simulink model "LaneMaintainSystem_Kavya"  (R2022b)
settings: Solver=VariableStepAuto  StartTime=0.0  StopTime=5  FixedStep=0.01  RelTol=1e-3
values from neighbouring files (symbols this model uses):
  A = [-0.5  -0.3  -0.01; 1  0  0; 0  1  0]    [kavya.mat]
  B = [1 0 0]    [kavya.mat]
  C = [0 0 1]    [kavya.mat]
  Ke = [2.00093781518 12.4255969567 11.1736830953]    [kavya.mat]
  Kr = [14.0661259067 105.961011965 9.990005]    [kavya.mat]
  uD = -0.1    [kavya.mat]
settings Model: Creator=abane  LastModifiedBy=chand

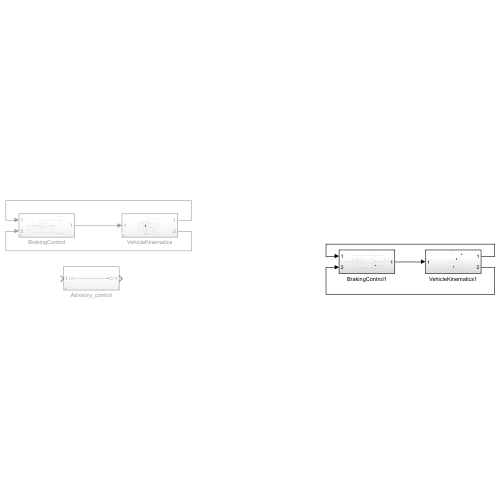
[thumbnail: Simulink's stored preview of the top-level diagram]
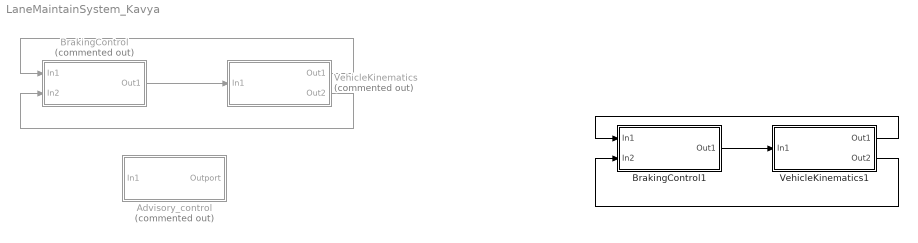
== system LaneMaintainSystem_Kavya ==
  Advisory_control : Subsystem  Commented=on
  BrakingControl : Subsystem  Commented=on
  BrakingControl1 : Subsystem
  VehicleKinematics : Subsystem  Commented=on
  VehicleKinematics1 : Subsystem
  wires:
  BrakingControl/1(Out1) -> VehicleKinematics/1(In1)
  VehicleKinematics/2(Out2) -> BrakingControl/2(In2)
  VehicleKinematics/1(Out1) -> BrakingControl/1(In1)
  BrakingControl1/1(Out1) -> VehicleKinematics1/1(In1)
  VehicleKinematics1/1(Out1) -> BrakingControl1/1(In1)
  VehicleKinematics1/2(Out2) -> BrakingControl1/2(In2)

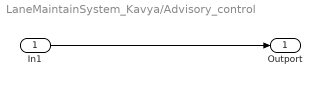
== system LaneMaintainSystem_Kavya/Advisory_control ==
  In1 : Inport
  Outport : Outport
  wires:
  In1/1 -> Outport/1

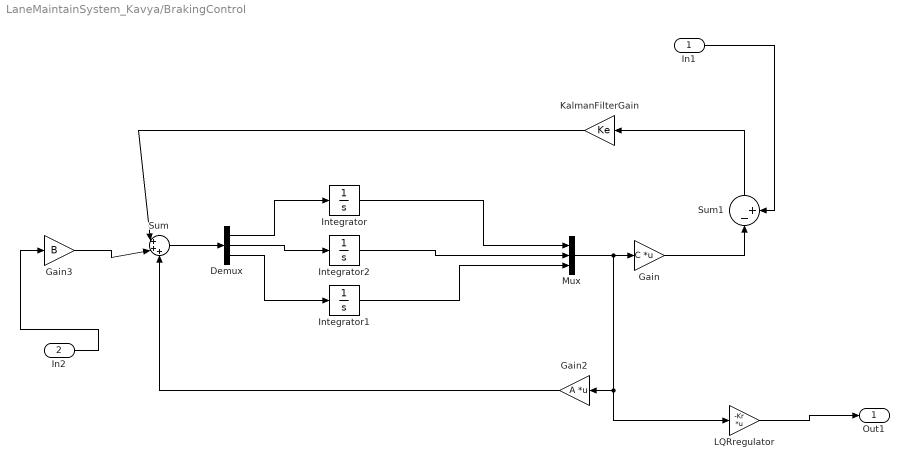
== system LaneMaintainSystem_Kavya/BrakingControl ==
  In1 : Inport
  In2 : Inport  Port=2
  Demux : Demux  Outputs=3
  Gain : Gain  Gain=C  Multiplication=Matrix(K*u)
  Gain2 : Gain  Gain=A  Multiplication=Matrix(K*u)
  Gain3 : Gain  Gain=B
  Integrator : Integrator
  Integrator1 : Integrator
  Integrator2 : Integrator
  KalmanFilterGain : Gain  Gain=Ke
  LQRregulator : Gain  Gain=-Kr  Multiplication=Matrix(K*u)
  Mux : Mux  Inputs=3
  Sum : Sum  Inputs=|+++
  Sum1 : Sum  Inputs=|-+
  Out1 : Outport
  wires:
  Sum/1 -> Demux/1
  Demux/1 -> Integrator/1
  Demux/3 -> Integrator1/1
  Integrator/1 -> Mux/1
  Integrator1/1 -> Mux/3
  Mux/1 -> LQRregulator/1, Gain2/1, Gain/1
  Gain/1 -> Sum1/1
  Sum1/1 -> KalmanFilterGain/1
  KalmanFilterGain/1 -> Sum/1
  Gain2/1 -> Sum/3
  Gain3/1 -> Sum/2
  LQRregulator/1 -> Out1/1
  In2/1 -> Gain3/1
  Demux/2 -> Integrator2/1
  Integrator2/1 -> Mux/2
  In1/1 -> Sum1/2

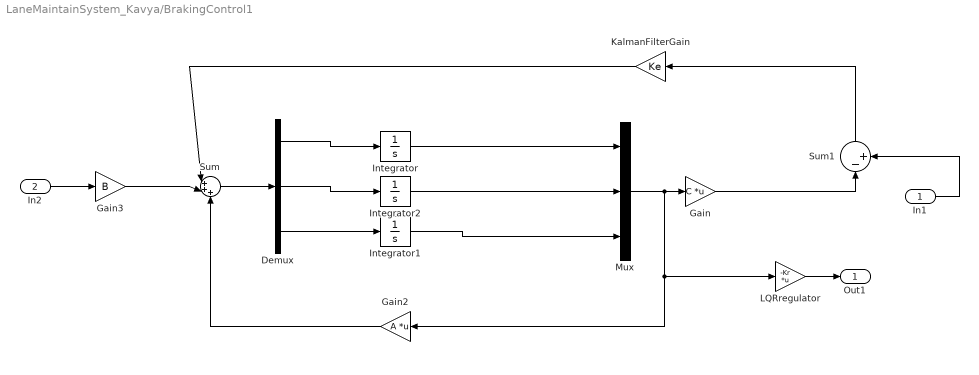
== system LaneMaintainSystem_Kavya/BrakingControl1 ==
  In1 : Inport
  In2 : Inport  Port=2
  Demux : Demux  Outputs=3
  Gain : Gain  Gain=C  Multiplication=Matrix(K*u)
  Gain2 : Gain  Gain=A  Multiplication=Matrix(K*u)
  Gain3 : Gain  Gain=B
  Integrator : Integrator
  Integrator1 : Integrator
  Integrator2 : Integrator
  KalmanFilterGain : Gain  Gain=Ke
  LQRregulator : Gain  Gain=-Kr  Multiplication=Matrix(K*u)
  Mux : Mux  Inputs=3
  Sum : Sum  Inputs=|+++
  Sum1 : Sum  Inputs=|-+
  Out1 : Outport
  wires:
  In1/1 -> Sum1/2
  Integrator2/1 -> Mux/2
  Demux/2 -> Integrator2/1
  In2/1 -> Gain3/1
  LQRregulator/1 -> Out1/1
  Gain3/1 -> Sum/2
  Gain2/1 -> Sum/3
  KalmanFilterGain/1 -> Sum/1
  Sum1/1 -> KalmanFilterGain/1
  Gain/1 -> Sum1/1
  Mux/1 -> Gain2/1, LQRregulator/1, Gain/1
  Integrator1/1 -> Mux/3
  Integrator/1 -> Mux/1
  Demux/3 -> Integrator1/1
  Demux/1 -> Integrator/1
  Sum/1 -> Demux/1

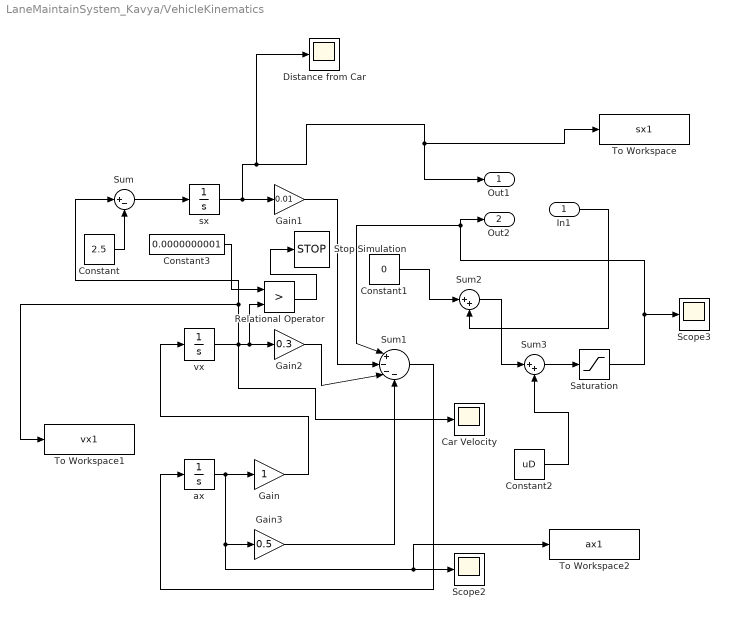
== system LaneMaintainSystem_Kavya/VehicleKinematics ==
  In1 : Inport
  Car Velocity : Scope
  Constant : Constant  Value=2.5
  Constant1 : Constant  Value=0
  Constant2 : Constant  Value=uD
  Constant3 : Constant  Value=0.0000000001
  Distance from Car : Scope
  Gain : Gain
  Gain1 : Gain  Gain=0.01
  Gain2 : Gain  Gain=0.3
  Gain3 : Gain  Gain=0.5
  Relational Operator : RelationalOperator  Operator=>  OutDataTypeStr=boolean  RndMeth=Simplest  InputSameDT=off
  Saturation : Saturate  UpperLimit=0  LowerLimit=-200
  Scope2 : Scope
  Scope3 : Scope
  Stop Simulation : Stop
  Sum : Sum  Inputs=|+-
  Sum1 : Sum  Inputs=|+---
  Sum2 : Sum  Inputs=|++
  Sum3 : Sum  Inputs=|++
  To Workspace : ToWorkspace  VariableName=sx1  SaveFormat=Timeseries  SampleTime=-1
  To Workspace1 : ToWorkspace  VariableName=vx1  SaveFormat=Timeseries  SampleTime=-1
  To Workspace2 : ToWorkspace  VariableName=ax1  SaveFormat=Timeseries  SampleTime=-1
  ax : Integrator
  sx : Integrator  InitialCondition=-43.8
  vx : Integrator  InitialCondition=41.2
  Out1 : Outport
  Out2 : Outport  Port=2
  wires:
  Constant/1 -> Sum/2
  Sum3/1 -> Saturation/1
  Constant2/1 -> Sum3/2
  Gain1/1 -> Sum1/2
  vx/1 -> Car Velocity/1, To Workspace1/1, Sum/1, Relational Operator/2, Gain2/1
  Saturation/1 -> Out2/1, Sum1/1, Scope3/1
  Gain3/1 -> Sum1/4
  Sum1/1 -> ax/1
  sx/1 -> Distance from Car/1, Out1/1, To Workspace/1, Gain1/1
  Sum2/1 -> Sum3/1
  ax/1 -> To Workspace2/1, Scope2/1, Gain3/1, Gain/1
  In1/1 -> Sum2/2
  Gain2/1 -> Sum1/3
  Constant1/1 -> Sum2/1
  Gain/1 -> vx/1
  Sum/1 -> sx/1
  Relational Operator/1 -> Stop Simulation/1
  Constant3/1 -> Relational Operator/1

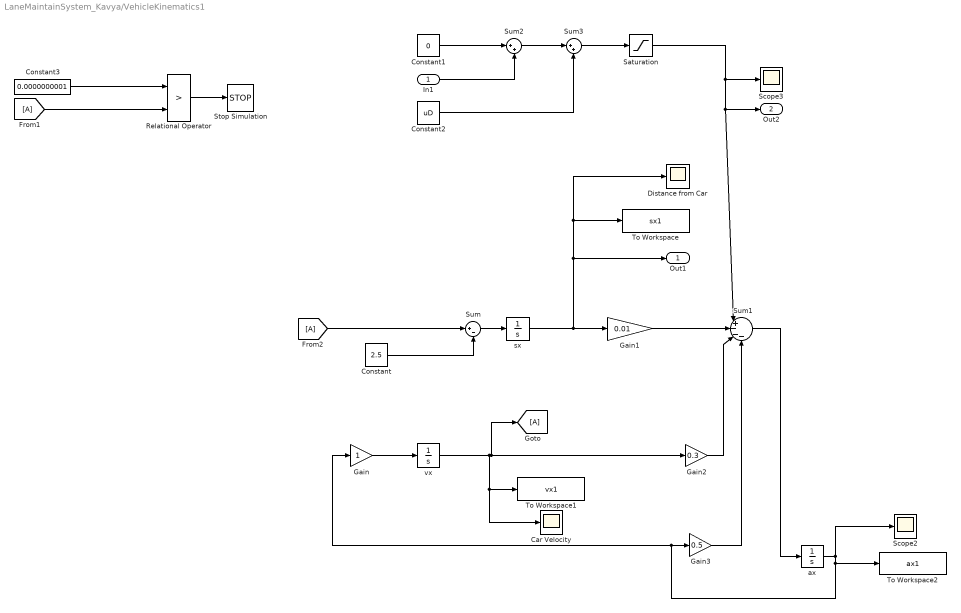
== system LaneMaintainSystem_Kavya/VehicleKinematics1 ==
  In1 : Inport
  Car Velocity : Scope
  Constant : Constant  Value=2.5
  Constant1 : Constant  Value=0
  Constant2 : Constant  Value=uD
  Constant3 : Constant  Value=0.0000000001
  Distance from Car : Scope
  From1 : From
  From2 : From
  Gain : Gain
  Gain1 : Gain  Gain=0.01
  Gain2 : Gain  Gain=0.3
  Gain3 : Gain  Gain=0.5
  Goto : Goto
  Relational Operator : RelationalOperator  Operator=>  OutDataTypeStr=boolean  RndMeth=Simplest  InputSameDT=off
  Saturation : Saturate  UpperLimit=0  LowerLimit=-300
  Scope2 : Scope
  Scope3 : Scope
  Stop Simulation : Stop
  Sum : Sum  Inputs=|+-
  Sum1 : Sum  Inputs=|+---
  Sum2 : Sum  Inputs=|++
  Sum3 : Sum  Inputs=|++
  To Workspace : ToWorkspace  VariableName=sx1  SampleTime=-1
  To Workspace1 : ToWorkspace  VariableName=vx1  SampleTime=-1
  To Workspace2 : ToWorkspace  VariableName=ax1  SampleTime=-1
  ax : Integrator
  sx : Integrator  InitialCondition=-43.8
  vx : Integrator  InitialCondition=41.2
  Out1 : Outport
  Out2 : Outport  Port=2
  wires:
  Constant3/1 -> Relational Operator/1
  Relational Operator/1 -> Stop Simulation/1
  Sum/1 -> sx/1
  Gain/1 -> vx/1
  Constant1/1 -> Sum2/1
  Gain2/1 -> Sum1/3
  In1/1 -> Sum2/2
  ax/1 -> To Workspace2/1, Gain/1, Gain3/1, Scope2/1
  Sum2/1 -> Sum3/1
  sx/1 -> Distance from Car/1, To Workspace/1, Out1/1, Gain1/1
  Sum1/1 -> ax/1
  Gain3/1 -> Sum1/4
  vx/1 -> Car Velocity/1, To Workspace1/1, Goto/1, Gain2/1
  Gain1/1 -> Sum1/2
  Constant2/1 -> Sum3/2
  Sum3/1 -> Saturation/1
  Constant/1 -> Sum/2
  Saturation/1 -> Sum1/1, Out2/1, Scope3/1
  From1/1 -> Relational Operator/2
  From2/1 -> Sum/1
